simulink model "tous"  (R2025a)
settings: Solver=VariableStepAuto  StartTime=0.0  StopTime=10.0  RelTol=1e-3
undefined symbols (not defined in the file or in its folder): stateSpaceParameters_1
libraries: hdlssclib x12, hdlsllib x10, library_AnalogOut x3, simulink x3
(part 1 of 2)
settings Model: Creator=bensa  LastModifiedBy=bensa

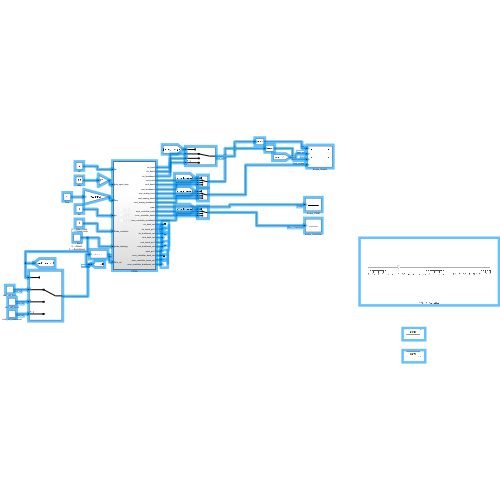
[thumbnail: Simulink's stored preview of the top-level diagram]
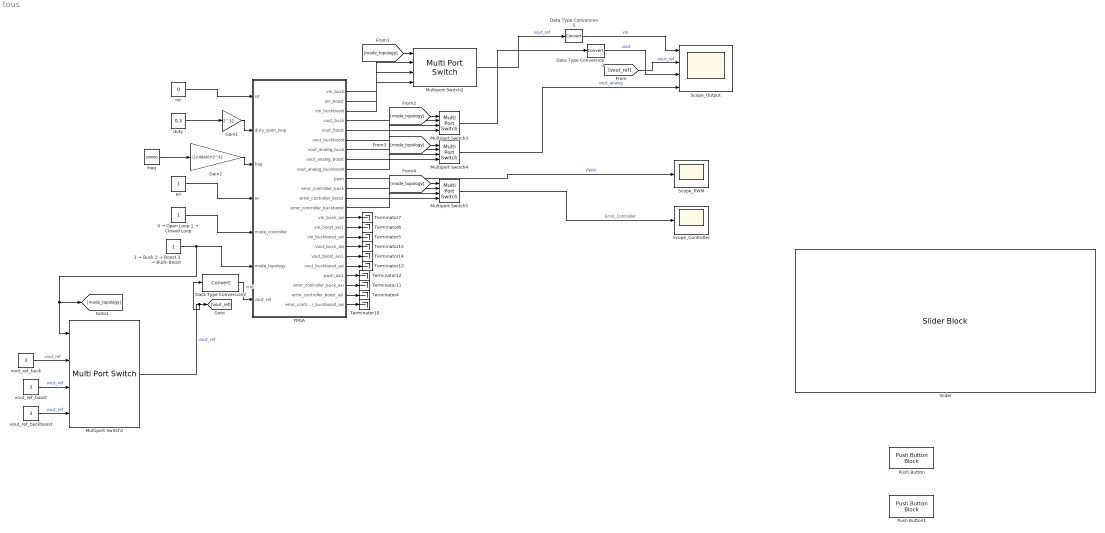
== system tous ==
  0 → Open Loop 1 → Closed Loop : Constant  OutDataTypeStr=uint32  SampleTime=25e-9
  1 → Buck 2 → Boost 3 → Buck-Boost : Constant  OutDataTypeStr=uint32  SampleTime=25e-9
  Data Type Conversion2 : DataTypeConversion  SaturateOnIntegerOverflow=off  RndMeth=Floor
  Data Type Conversion3 : DataTypeConversion  RndMeth=Nearest  SaturateOnIntegerOverflow=off  LockScale=on
  Data Type Conversion5 : DataTypeConversion  RndMeth=Nearest  SaturateOnIntegerOverflow=off  LockScale=on
  FPGA : Subsystem  TreatAsAtomicUnit=on
  Gain1 : Gain  Gain=2^32  OutDataTypeStr=uint32
  Gain2 : Gain  Gain=(1/(40e6))*2^32  OutDataTypeStr=uint32
  Multiport Switch{1..5} (5 alike) : MultiPortSwitch  SaturateOnIntegerOverflow=off  InputSameDT=off
  Push Button : PushButtonBlock  IconOnColor=[0.0, 0.39215686274509803, 0.0]  IconOffColor=[0.0, 1.0, 0.0]
  Push Button1 : PushButtonBlock  IconOnColor=[0.0, 0.39215686274509803, 0.0]  IconOffColor=[0.0, 1.0, 0.0]
  Scope_Controller : Scope
      settings: ActiveDisplayYMinimum=-13.875  ActiveDisplayYMaximum=24.875  DataLoggingVariableName=ScopeData3
  Scope_Output : Scope  NumInputPorts=4
      settings: ActiveDisplayYMinimum=-1.4999999999999996  ActiveDisplayYMaximum=13.5
  Scope_PWM : Scope
      settings: ActiveDisplayYMinimum=-0.62499999999999989  ActiveDisplayYMaximum=5.625
  Slider : SliderBlock  LabelPosition=Bottom  ScaleMax=12
  Terminator{4..7,10..15} (10 alike) : Terminator
  duty : Constant  Value=0.3  OutDataTypeStr=double  SampleTime=25e-9
  en : Constant  OutDataTypeStr=uint32  SampleTime=25e-9
  freq : Constant  Value=100000  SampleTime=25e-9
  rst : Constant  Value=0  OutDataTypeStr=uint32  SampleTime=25e-9
  vout_ref_boost : Constant  Value=3  OutDataTypeStr=double  SampleTime=25e-9
  vout_ref_buck : Constant  Value=3  OutDataTypeStr=double  SampleTime=25e-9
  vout_ref_buckboost : Constant  Value=3  OutDataTypeStr=double  SampleTime=25e-9
  wires:
  duty/1 -> Gain1/1
  [vout_ref] -> Scope_Output/2  "vout_ref"
  FPGA/7(vout_analog_buck) -> Multiport Switch4/2
  FPGA/14(vin_buck_axi) -> Terminator7/1
  FPGA/5(vout_boost) -> Multiport Switch3/3
  FPGA/4(vout_buck) -> Multiport Switch3/2
  0 → Open Loop 1 → Closed Loop/1 -> FPGA/5(mode_controller)
  1 → Buck 2 → Boost 3 → Buck-Boost/1 -> FPGA/6(mode_topology), [mode_topology], Multiport Switch1/1
  FPGA/22(error_controller_boost_axi) -> Terminator4/1
  FPGA/12(error_controller_boost) -> Multiport Switch5/3
  Data Type Conversion3/1 -> Scope_Output/3  "vout"
  FPGA/2(vin_boost) -> Multiport Switch2/3
  FPGA/11(error_controller_buck) -> Multiport Switch5/2
  FPGA/13(error_controller_buckboost) -> Multiport Switch5/4
  vout_ref_buck/1 -> Multiport Switch1/2  "vout_ref"
  FPGA/21(error_controller_buck_axi) -> Terminator11/1
  [mode_topology] -> Multiport Switch2/1
  FPGA/16(vin_buckboost_axi) -> Terminator5/1
  FPGA/10(pwm) -> Scope_PWM/1  "PWM"
  rst/1 -> FPGA/1(rst)
  Multiport Switch4/1 -> Scope_Output/4  "vout_analog"
  FPGA/17(vout_buck_axi) -> Terminator15/1
  FPGA/9(vout_analog_buckboost) -> Multiport Switch4/4
  freq/1 -> Gain2/1
  Multiport Switch5/1 -> Scope_Controller/1  "Error_Controller"
  Multiport Switch2/1 -> Data Type Conversion5/1  "vout_ref"
  FPGA/6(vout_buckboost) -> Multiport Switch3/4
  Gain1/1 -> FPGA/2(duty_open_loop)
  Multiport Switch1/1 -> Data Type Conversion2/1, [vout_ref]  "vout_ref"
  FPGA/23(error_controller_buckboost_axi) -> Terminator10/1
  Data Type Conversion2/1 -> FPGA/7(vout_ref)  "vref"
  [mode_topology] -> Multiport Switch5/1
  vout_ref_buckboost/1 -> Multiport Switch1/4  "vout_ref"
  vout_ref_boost/1 -> Multiport Switch1/3  "vout_ref"
  FPGA/1(vin_buck) -> Multiport Switch2/2
  Data Type Conversion5/1 -> Scope_Output/1  "vin"
  en/1 -> FPGA/4(en)
  FPGA/8(vout_analog_boost) -> Multiport Switch4/3
  [mode_topology] -> Multiport Switch3/1
  FPGA/19(vout_buckboost_axi) -> Terminator13/1
  FPGA/18(vout_boost_axi1) -> Terminator14/1
  Gain2/1 -> FPGA/3(freq)
  Multiport Switch3/1 -> Data Type Conversion3/1
  [mode_topology] -> Multiport Switch4/1
  FPGA/20(pwm_axi1) -> Terminator12/1
  FPGA/3(vin_buckboost) -> Multiport Switch2/4
  FPGA/15(vin_boost_axi1) -> Terminator6/1

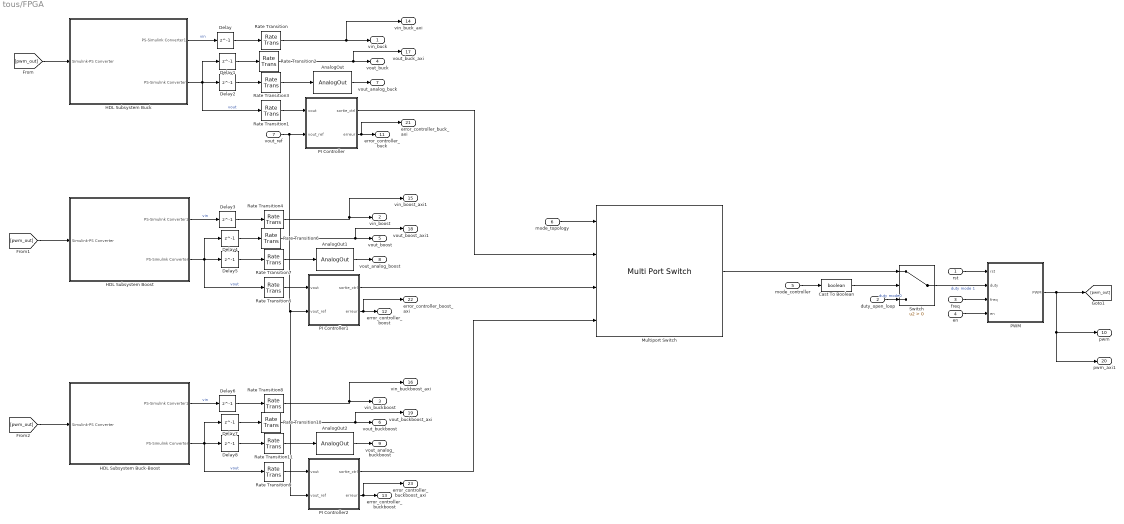
== system tous/FPGA ==
  rst : Inport  OutDataTypeStr=uint32
  duty_open_loop : Inport  Port=2  OutDataTypeStr=uint32
  freq : Inport  Port=3  OutDataTypeStr=uint32
  en : Inport  Port=4  OutDataTypeStr=uint32
  mode_controller : Inport  Port=5  OutDataTypeStr=uint32
  mode_topology : Inport  Port=6
  vout_ref : Inport  Port=7  OutDataTypeStr=uint32
  AnalogOut : library_AnalogOut/AnalogOut  SignalMin=0  SignalMax=12  VoltageMin=0  VoltageMax=4
  AnalogOut1 : library_AnalogOut/AnalogOut  SignalMin=0  SignalMax=12  VoltageMin=0  VoltageMax=4
  AnalogOut2 : library_AnalogOut/AnalogOut  SignalMin=0  SignalMax=12  VoltageMin=0  VoltageMax=4
  Cast To Boolean : DataTypeConversion  OutDataTypeStr=boolean  SaturateOnIntegerOverflow=off  RndMeth=Floor
  Delay{,1..8} (9 alike) : Delay  DelayLength=1
  HDL Subsystem Boost : Subsystem  DataTypeOverride=Off  MinMaxOverflowLogging=MinMaxAndOverflow
  HDL Subsystem Buck : Subsystem  DataTypeOverride=Off  MinMaxOverflowLogging=MinMaxAndOverflow
  HDL Subsystem Buck-Boost : Subsystem  DataTypeOverride=Off  MinMaxOverflowLogging=MinMaxAndOverflow
  Multiport Switch : MultiPortSwitch  SaturateOnIntegerOverflow=off  InputSameDT=off
  PI Controller : Subsystem
  PI Controller1 : Subsystem
  PI Controller2 : Subsystem
  PWM : Subsystem
  Rate Transition{,2..4,6..8,10..11} (9 alike) : RateTransition  OutPortSampleTime=25e-9
  Rate Transition1 : RateTransition
  Rate Transition5 : RateTransition
  Rate Transition9 : RateTransition
  Switch : Switch  Criteria=u2 > Threshold  SaturateOnIntegerOverflow=off  InputSameDT=off
  vin_buck : Outport
  vin_boost : Outport  Port=2
  vin_buckboost : Outport  Port=3
  vout_buck : Outport  Port=4
  vout_boost : Outport  Port=5
  vout_buckboost : Outport  Port=6
  vout_analog_buck : Outport  Port=7
  vout_analog_boost : Outport  Port=8
  vout_analog_buckboost : Outport  Port=9
  pwm : Outport  Port=10
  error_controller_buck : Outport  Port=11
  error_controller_boost : Outport  Port=12
  error_controller_buckboost : Outport  Port=13
  vin_buck_axi : Outport  Port=14
  vin_boost_axi1 : Outport  Port=15
  vin_buckboost_axi : Outport  Port=16
  vout_buck_axi : Outport  Port=17
  vout_boost_axi1 : Outport  Port=18
  vout_buckboost_axi : Outport  Port=19
  pwm_axi1 : Outport  Port=20
  error_controller_buck_axi : Outport  Port=21
  error_controller_boost_axi : Outport  Port=22
  error_controller_buckboost_axi : Outport  Port=23
  wires:
  HDL Subsystem Buck/1(PS-Simulink Converter1) -> Delay/1  "vin"
  HDL Subsystem Buck/2(PS-Simulink Converter) -> Rate Transition1/1, Delay2/1, Delay1/1  "vout"
  Delay1/1 -> Rate Transition2/1
  Delay/1 -> Rate Transition/1
  Rate Transition2/1 -> vout_buck_axi/1, vout_buck/1
  Rate Transition/1 -> vin_buck_axi/1, vin_buck/1
  AnalogOut/1 -> vout_analog_buck/1
  PI Controller/2(erreur) -> error_controller_buck_axi/1, error_controller_buck/1
  Rate Transition1/1 -> PI Controller/1(vout)
  Delay2/1 -> Rate Transition3/1
  Rate Transition3/1 -> AnalogOut/1
  PI Controller/1(sortie_ctrl) -> Multiport Switch/2
  mode_topology/1 -> Multiport Switch/1
  Delay4/1 -> Rate Transition6/1
  Rate Transition7/1 -> AnalogOut1/1
  Delay3/1 -> Rate Transition4/1
  PI Controller1/2(erreur) -> error_controller_boost_axi/1, error_controller_boost/1
  PI Controller1/1(sortie_ctrl) -> Multiport Switch/3
  HDL Subsystem Boost/1(PS-Simulink Converter1) -> Delay3/1  "vin"
  HDL Subsystem Boost/2(PS-Simulink Converter) -> Rate Transition5/1, Delay5/1, Delay4/1  "vout"
  Rate Transition6/1 -> vout_boost_axi1/1, vout_boost/1
  Rate Transition5/1 -> PI Controller1/1(vout)
  Rate Transition4/1 -> vin_boost_axi1/1, vin_boost/1
  Delay5/1 -> Rate Transition7/1
  AnalogOut1/1 -> vout_analog_boost/1
  vout_ref/1 -> PI Controller2/2(vout_ref), PI Controller1/2(vout_ref), PI Controller/2(vout_ref)
  Delay7/1 -> Rate Transition10/1
  Rate Transition11/1 -> AnalogOut2/1
  Delay6/1 -> Rate Transition8/1
  PI Controller2/2(erreur) -> error_controller_buckboost_axi/1, error_controller_buckboost/1
  PI Controller2/1(sortie_ctrl) -> Multiport Switch/4
  HDL Subsystem Buck-Boost/1(PS-Simulink Converter1) -> Delay6/1  "vin"
  HDL Subsystem Buck-Boost/2(PS-Simulink Converter) -> Rate Transition9/1, Delay8/1, Delay7/1  "vout"
  Rate Transition10/1 -> vout_buckboost_axi/1, vout_buckboost/1
  Rate Transition9/1 -> PI Controller2/1(vout)
  Rate Transition8/1 -> vin_buckboost_axi/1, vin_buckboost/1
  Delay8/1 -> Rate Transition11/1
  AnalogOut2/1 -> vout_analog_buckboost/1
  Multiport Switch/1 -> Switch/1
  Switch/1 -> PWM/2(duty)  "duty mode 1"
  duty_open_loop/1 -> Switch/3  "duty mode0"
  freq/1 -> PWM/3(freq)
  rst/1 -> PWM/1(rst)
  en/1 -> PWM/4(en)
  Cast To Boolean/1 -> Switch/2
  mode_controller/1 -> Cast To Boolean/1
  PWM/1(PWM) -> pwm/1, pwm_axi1/1, [pwm_out]
  [pwm_out] -> HDL Subsystem Buck/1(Simulink-PS Converter)
  [pwm_out] -> HDL Subsystem Boost/1(Simulink-PS Converter)
  [pwm_out] -> HDL Subsystem Buck-Boost/1(Simulink-PS Converter)

== system tous/FPGA/HDL Subsystem Boost ==
  Simulink-PS Converter : Inport  OutDataTypeStr=fixdt(0,32,29)
  HDL Algorithm : Subsystem
  Input Concat : Concatenate  NumInputs=1
  Output Demux : Demux  Outputs=2
  Rate Transition2 : RateTransition  Integrity=off  OutPortSampleTimeOpt=Multiple of input port sample time  OutPortSampleTimeMultiple=1/2
  Rate Transition3 : RateTransition  OutPortSampleTimeOpt=Multiple of input port sample time  OutPortSampleTimeMultiple=2
  Rate Transition4 : RateTransition  OutPortSampleTimeOpt=Multiple of input port sample time  OutPortSampleTimeMultiple=2
  Valid Out : Terminator
  PS-Simulink Converter1 : Outport
  PS-Simulink Converter : Outport  Port=2
  wires:
  HDL Algorithm/1(Out1) -> Output Demux/1
  Rate Transition3/1 -> PS-Simulink Converter1/1  "PS-Simulink Converter1"
  HDL Algorithm/2(Valid Out) -> Valid Out/1
  Output Demux/2 -> Rate Transition4/1
  Output Demux/1 -> Rate Transition3/1
  Simulink-PS Converter/1 -> Rate Transition2/1
  Input Concat/1 -> HDL Algorithm/1(In1)
  Rate Transition2/1 -> Input Concat/1
  Rate Transition4/1 -> PS-Simulink Converter/1  "PS-Simulink Converter"

== system tous/FPGA/HDL Subsystem Buck ==
  Simulink-PS Converter : Inport  OutDataTypeStr=fixdt(0,32,29)
  HDL Algorithm : Subsystem
  Input Concat : Concatenate  NumInputs=1
  Output Demux : Demux  Outputs=2
  Rate Transition2 : RateTransition  Integrity=off  OutPortSampleTimeOpt=Multiple of input port sample time  OutPortSampleTimeMultiple=1/2
  Rate Transition3 : RateTransition  OutPortSampleTimeOpt=Multiple of input port sample time  OutPortSampleTimeMultiple=2
  Rate Transition4 : RateTransition  OutPortSampleTimeOpt=Multiple of input port sample time  OutPortSampleTimeMultiple=2
  Valid Out : Terminator
  PS-Simulink Converter1 : Outport
  PS-Simulink Converter : Outport  Port=2
  wires:
  Output Demux/2 -> Rate Transition4/1
  Rate Transition3/1 -> PS-Simulink Converter1/1  "PS-Simulink Converter1"
  HDL Algorithm/2(Valid Out) -> Valid Out/1
  Input Concat/1 -> HDL Algorithm/1(In1)
  Output Demux/1 -> Rate Transition3/1
  Simulink-PS Converter/1 -> Rate Transition2/1
  HDL Algorithm/1(Out1) -> Output Demux/1
  Rate Transition4/1 -> PS-Simulink Converter/1  "PS-Simulink Converter"
  Rate Transition2/1 -> Input Concat/1

== system tous/FPGA/HDL Subsystem Buck-Boost ==
  Simulink-PS Converter : Inport  OutDataTypeStr=fixdt(0,32,29)
  HDL Algorithm : Subsystem
  Input Concat : Concatenate  NumInputs=1
  Output Demux : Demux  Outputs=2
  Rate Transition2 : RateTransition  Integrity=off  OutPortSampleTimeOpt=Multiple of input port sample time  OutPortSampleTimeMultiple=1/2
  Rate Transition3 : RateTransition  OutPortSampleTimeOpt=Multiple of input port sample time  OutPortSampleTimeMultiple=2
  Rate Transition4 : RateTransition  OutPortSampleTimeOpt=Multiple of input port sample time  OutPortSampleTimeMultiple=2
  Valid Out : Terminator
  PS-Simulink Converter1 : Outport
  PS-Simulink Converter : Outport  Port=2
  wires:
  Rate Transition3/1 -> PS-Simulink Converter1/1  "PS-Simulink Converter1"
  Rate Transition2/1 -> Input Concat/1
  Input Concat/1 -> HDL Algorithm/1(In1)
  Simulink-PS Converter/1 -> Rate Transition2/1
  Output Demux/1 -> Rate Transition3/1
  Rate Transition4/1 -> PS-Simulink Converter/1  "PS-Simulink Converter"
  Output Demux/2 -> Rate Transition4/1
  HDL Algorithm/1(Out1) -> Output Demux/1
  HDL Algorithm/2(Valid Out) -> Valid Out/1

== system tous/FPGA/PI Controller ==
  vout : Inport
  vout_ref : Inport  Port=2  OutDataTypeStr=uint32
  Controller : Subsystem
  Data Type Conversion : DataTypeConversion  SaturateOnIntegerOverflow=off  RndMeth=Floor
  Data Type Conversion1 : DataTypeConversion  SaturateOnIntegerOverflow=off  RndMeth=Floor
  Data Type Conversion2 : DataTypeConversion  SaturateOnIntegerOverflow=off  RndMeth=Floor
  Gain3 : Gain  Gain=2^32  OutDataTypeStr=uint32
  ki : Constant  Value=3.07e-80  OutDataTypeStr=double  SampleTime=25e-9
  kp : Constant  Value=3  OutDataTypeStr=double  SampleTime=25e-9
  sortie_ctrl : Outport
  erreur : Outport  Port=2
  wires:
  vout/1 -> Data Type Conversion/1
  Controller/1(sortie_ctrl) -> Gain3/1
  Data Type Conversion1/1 -> Controller/3(kp)
  kp/1 -> Data Type Conversion1/1
  ki/1 -> Data Type Conversion2/1
  vout_ref/1 -> Controller/1(vout_ref)
  Data Type Conversion/1 -> Controller/2(vout)
  Data Type Conversion2/1 -> Controller/4(ki)
  Gain3/1 -> sortie_ctrl/1
  Controller/2(error_ctrl) -> erreur/1

== system tous/FPGA/PI Controller1 ==
  vout : Inport
  vout_ref : Inport  Port=2  OutDataTypeStr=uint32
  Controller : Subsystem
  Data Type Conversion : DataTypeConversion  SaturateOnIntegerOverflow=off  RndMeth=Floor
  Data Type Conversion1 : DataTypeConversion  SaturateOnIntegerOverflow=off  RndMeth=Floor
  Data Type Conversion2 : DataTypeConversion  SaturateOnIntegerOverflow=off  RndMeth=Floor
  Gain3 : Gain  Gain=2^32  OutDataTypeStr=uint32
  ki : Constant  Value=3.07e-80  OutDataTypeStr=double  SampleTime=25e-9
  kp : Constant  Value=3  OutDataTypeStr=double  SampleTime=25e-9
  sortie_ctrl : Outport
  erreur : Outport  Port=2
  wires:
  vout/1 -> Data Type Conversion/1
  Controller/1(sortie_ctrl) -> Gain3/1
  Data Type Conversion1/1 -> Controller/3(kp)
  kp/1 -> Data Type Conversion1/1
  ki/1 -> Data Type Conversion2/1
  vout_ref/1 -> Controller/1(vout_ref)
  Data Type Conversion/1 -> Controller/2(vout)
  Data Type Conversion2/1 -> Controller/4(ki)
  Gain3/1 -> sortie_ctrl/1
  Controller/2(error_ctrl) -> erreur/1

== system tous/FPGA/PI Controller2 ==
  vout : Inport
  vout_ref : Inport  Port=2  OutDataTypeStr=uint32
  Controller : Subsystem
  Data Type Conversion : DataTypeConversion  SaturateOnIntegerOverflow=off  RndMeth=Floor
  Data Type Conversion1 : DataTypeConversion  SaturateOnIntegerOverflow=off  RndMeth=Floor
  Data Type Conversion2 : DataTypeConversion  SaturateOnIntegerOverflow=off  RndMeth=Floor
  Gain3 : Gain  Gain=2^32  OutDataTypeStr=uint32
  ki : Constant  Value=3.07e-80  OutDataTypeStr=double  SampleTime=25e-9
  kp : Constant  Value=3  OutDataTypeStr=double  SampleTime=25e-9
  sortie_ctrl : Outport
  erreur : Outport  Port=2
  wires:
  vout/1 -> Data Type Conversion/1
  Controller/1(sortie_ctrl) -> Gain3/1
  Data Type Conversion1/1 -> Controller/3(kp)
  kp/1 -> Data Type Conversion1/1
  ki/1 -> Data Type Conversion2/1
  vout_ref/1 -> Controller/1(vout_ref)
  Data Type Conversion/1 -> Controller/2(vout)
  Data Type Conversion2/1 -> Controller/4(ki)
  Gain3/1 -> sortie_ctrl/1
  Controller/2(error_ctrl) -> erreur/1

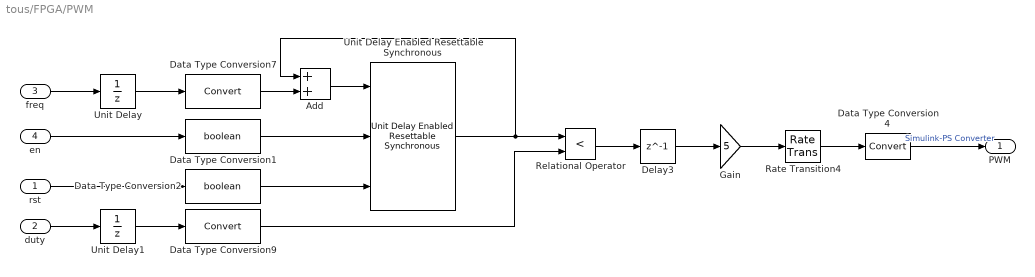
== system tous/FPGA/PWM ==
  rst : Inport  OutDataTypeStr=uint32
  duty : Inport  Port=2  OutDataTypeStr=uint32
  freq : Inport  Port=3  OutDataTypeStr=uint32
  en : Inport  Port=4  OutDataTypeStr=uint32
  Add : Sum  OutDataTypeStr=uint32  AccumDataTypeStr=uint32
  Data Type Conversion1 : DataTypeConversion  OutDataTypeStr=boolean  SaturateOnIntegerOverflow=off  RndMeth=Floor
  Data Type Conversion2 : DataTypeConversion  OutDataTypeStr=boolean  SaturateOnIntegerOverflow=off  RndMeth=Floor
  Data Type Conversion4 : DataTypeConversion  RndMeth=Nearest  SaturateOnIntegerOverflow=off
  Data Type Conversion7 : DataTypeConversion  SaturateOnIntegerOverflow=off  RndMeth=Floor
  Data Type Conversion9 : DataTypeConversion  SaturateOnIntegerOverflow=off  RndMeth=Floor
  Delay3 : Delay  DelayLength=1
  Gain : Gain  Gain=5
  Rate Transition4 : RateTransition  OutPortSampleTime=5e-08
  Relational Operator : RelationalOperator  Operator=<  OutDataTypeStr=boolean  RndMeth=Simplest  InputSameDT=off
  Unit Delay : UnitDelay  SampleTime=-1  HasFrameUpgradeWarning=on
  Unit Delay Enabled Resettable Synchronous : hdlsllib/Discrete/Unit Delay Enabled Resettable Synchronous  InitialCondition=0.0  SampleTime=-1
  Unit Delay1 : UnitDelay  SampleTime=-1  HasFrameUpgradeWarning=on
  PWM : Outport
  wires:
  Rate Transition4/1 -> Data Type Conversion4/1
  en/1 -> Data Type Conversion1/1
  Data Type Conversion1/1 -> Unit Delay Enabled Resettable Synchronous/2
  Unit Delay/1 -> Data Type Conversion7/1
  Data Type Conversion7/1 -> Add/2
  Gain/1 -> Rate Transition4/1
  Delay3/1 -> Gain/1
  Data Type Conversion2/1 -> Unit Delay Enabled Resettable Synchronous/3
  Add/1 -> Unit Delay Enabled Resettable Synchronous/1
  freq/1 -> Unit Delay/1
  Unit Delay Enabled Resettable Synchronous/1 -> Add/1, Relational Operator/1
  Unit Delay1/1 -> Data Type Conversion9/1
  rst/1 -> Data Type Conversion2/1
  Data Type Conversion9/1 -> Relational Operator/2
  Relational Operator/1 -> Delay3/1
  duty/1 -> Unit Delay1/1
  Data Type Conversion4/1 -> PWM/1  "Simulink-PS Converter"

== system tous/FPGA/HDL Subsystem Boost/HDL Algorithm ==
  In1 : Inport  OutDataTypeStr=fixdt(0,32,29)
  Delay : Delay  DelayLength=1
  Delay1 : Delay
  Mode Iteration Manager : Subsystem
  Mode Selection : Subsystem
  Output : Subsystem
  State Delay : Delay  DelayLength=1  InitialCondition=single(stateSpaceParameters_1.X0)
  State Update : Subsystem
  Out1 : Outport  VectorParamsAs1DForOutWhenUnconnected=off
  Valid Out : Outport  Port=2  VectorParamsAs1DForOutWhenUnconnected=off
  wires:
  In1/1 -> Mode Selection/1(In1), Delay1/1, State Update/1(In1)
  Delay1/1 -> Output/1(In1)
  State Update/1(State Out) -> State Delay/1
  Mode Selection/1(Out1) -> Mode Iteration Manager/2(In2)
  State Delay/1 -> Mode Iteration Manager/1(In1), Mode Selection/2(In2)
  Delay/1 -> Output/3(Sel)
  Mode Iteration Manager/1(Out1) -> State Update/2(State), Output/2(State)
  Mode Selection/2(Out2) -> Delay/1
  Mode Iteration Manager/2(Out2) -> State Update/3(Sel)
  Mode Iteration Manager/3(Valid Out) -> Valid Out/1
  Output/1(Out1) -> Out1/1

== system tous/FPGA/HDL Subsystem Buck/HDL Algorithm ==
  In1 : Inport  OutDataTypeStr=fixdt(0,32,29)
  Delay : Delay  DelayLength=1
  Delay1 : Delay
  Mode Iteration Manager : Subsystem
  Mode Selection : Subsystem
  Output : Subsystem
  State Delay : Delay  DelayLength=1  InitialCondition=single(stateSpaceParameters_1.X0)
  State Update : Subsystem
  Out1 : Outport  VectorParamsAs1DForOutWhenUnconnected=off
  Valid Out : Outport  Port=2  VectorParamsAs1DForOutWhenUnconnected=off
  wires:
  In1/1 -> Mode Selection/1(In1), Delay1/1, State Update/1(In1)
  State Update/1(State Out) -> State Delay/1
  Delay1/1 -> Output/1(In1)
  Mode Selection/2(Out2) -> Delay/1
  State Delay/1 -> Mode Iteration Manager/1(In1), Mode Selection/2(In2)
  Mode Selection/1(Out1) -> Mode Iteration Manager/2(In2)
  Delay/1 -> Output/3(Sel)
  Mode Iteration Manager/1(Out1) -> State Update/2(State), Output/2(State)
  Mode Iteration Manager/2(Out2) -> State Update/3(Sel)
  Mode Iteration Manager/3(Valid Out) -> Valid Out/1
  Output/1(Out1) -> Out1/1

== system tous/FPGA/HDL Subsystem Buck-Boost/HDL Algorithm ==
  In1 : Inport  OutDataTypeStr=fixdt(0,32,29)
  Delay : Delay  DelayLength=1
  Delay1 : Delay
  Mode Iteration Manager : Subsystem
  Mode Selection : Subsystem
  Output : Subsystem
  State Delay : Delay  DelayLength=1  InitialCondition=single(stateSpaceParameters_1.X0)
  State Update : Subsystem
  Out1 : Outport  VectorParamsAs1DForOutWhenUnconnected=off
  Valid Out : Outport  Port=2  VectorParamsAs1DForOutWhenUnconnected=off
  wires:
  In1/1 -> Mode Selection/1(In1), Delay1/1, State Update/1(In1)
  Delay/1 -> Output/3(Sel)
  Mode Selection/1(Out1) -> Mode Iteration Manager/2(In2)
  State Update/1(State Out) -> State Delay/1
  Delay1/1 -> Output/1(In1)
  Mode Selection/2(Out2) -> Delay/1
  Mode Iteration Manager/1(Out1) -> State Update/2(State), Output/2(State)
  State Delay/1 -> Mode Iteration Manager/1(In1), Mode Selection/2(In2)
  Mode Iteration Manager/2(Out2) -> State Update/3(Sel)
  Mode Iteration Manager/3(Valid Out) -> Valid Out/1
  Output/1(Out1) -> Out1/1

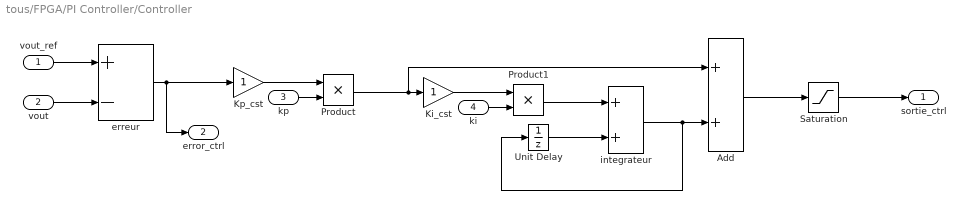
== system tous/FPGA/PI Controller/Controller ==
  vout_ref : Inport
  vout : Inport  Port=2
  kp : Inport  Port=3
  ki : Inport  Port=4
  Add : Sum  OutDataTypeStr=fixdt(1,32,25)  AccumDataTypeStr=fixdt(1,32,25)
  Ki_cst : Gain  OutDataTypeStr=fixdt(1,32,25)
  Kp_cst : Gain  OutDataTypeStr=fixdt(1,32,25)
  Product : Product
  Product1 : Product
  Saturation : Saturate  UpperLimit=0.95  LowerLimit=0.05  LinearizeAsGain=off
  Unit Delay : UnitDelay  SampleTime=-1  HasFrameUpgradeWarning=on
  erreur : Sum  Inputs=+-  OutDataTypeStr=fixdt(1,32,25)  AccumDataTypeStr=fixdt(1,32,25)
  integrateur : Sum  OutDataTypeStr=fixdt(1,32,25)  AccumDataTypeStr=fixdt(1,32,25)
  sortie_ctrl : Outport
  error_ctrl : Outport  Port=2
  wires:
  vout/1 -> erreur/2
  vout_ref/1 -> erreur/1
  integrateur/1 -> Unit Delay/1, Add/2
  erreur/1 -> error_ctrl/1, Kp_cst/1
  ki/1 -> Product1/2
  Ki_cst/1 -> Product1/1
  Kp_cst/1 -> Product/1
  Product/1 -> Add/1, Ki_cst/1
  kp/1 -> Product/2
  Product1/1 -> integrateur/1
  Add/1 -> Saturation/1
  Saturation/1 -> sortie_ctrl/1
  Unit Delay/1 -> integrateur/2

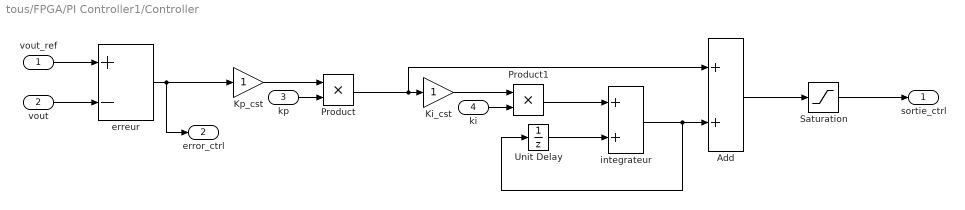
== system tous/FPGA/PI Controller1/Controller ==
  vout_ref : Inport
  vout : Inport  Port=2
  kp : Inport  Port=3
  ki : Inport  Port=4
  Add : Sum  OutDataTypeStr=fixdt(1,32,25)  AccumDataTypeStr=fixdt(1,32,25)
  Ki_cst : Gain  OutDataTypeStr=fixdt(1,32,25)
  Kp_cst : Gain  OutDataTypeStr=fixdt(1,32,25)
  Product : Product
  Product1 : Product
  Saturation : Saturate  UpperLimit=0.95  LowerLimit=0.05  LinearizeAsGain=off
  Unit Delay : UnitDelay  SampleTime=-1  HasFrameUpgradeWarning=on
  erreur : Sum  Inputs=+-  OutDataTypeStr=fixdt(1,32,25)  AccumDataTypeStr=fixdt(1,32,25)
  integrateur : Sum  OutDataTypeStr=fixdt(1,32,25)  AccumDataTypeStr=fixdt(1,32,25)
  sortie_ctrl : Outport
  error_ctrl : Outport  Port=2
  wires:
  vout/1 -> erreur/2
  vout_ref/1 -> erreur/1
  integrateur/1 -> Unit Delay/1, Add/2
  erreur/1 -> error_ctrl/1, Kp_cst/1
  ki/1 -> Product1/2
  Ki_cst/1 -> Product1/1
  Kp_cst/1 -> Product/1
  Product/1 -> Add/1, Ki_cst/1
  kp/1 -> Product/2
  Product1/1 -> integrateur/1
  Add/1 -> Saturation/1
  Saturation/1 -> sortie_ctrl/1
  Unit Delay/1 -> integrateur/2

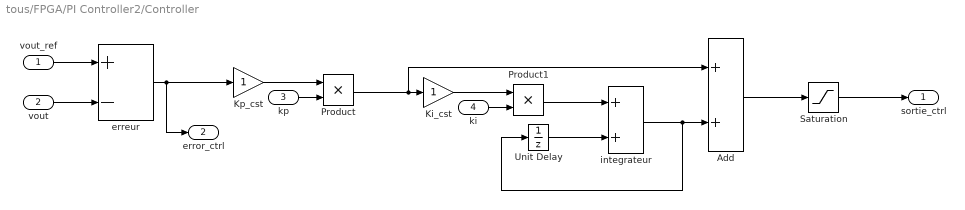
== system tous/FPGA/PI Controller2/Controller ==
  vout_ref : Inport
  vout : Inport  Port=2
  kp : Inport  Port=3
  ki : Inport  Port=4
  Add : Sum  OutDataTypeStr=fixdt(1,32,25)  AccumDataTypeStr=fixdt(1,32,25)
  Ki_cst : Gain  OutDataTypeStr=fixdt(1,32,25)
  Kp_cst : Gain  OutDataTypeStr=fixdt(1,32,25)
  Product : Product
  Product1 : Product
  Saturation : Saturate  UpperLimit=0.95  LowerLimit=0.05  LinearizeAsGain=off
  Unit Delay : UnitDelay  SampleTime=-1  HasFrameUpgradeWarning=on
  erreur : Sum  Inputs=+-  OutDataTypeStr=fixdt(1,32,25)  AccumDataTypeStr=fixdt(1,32,25)
  integrateur : Sum  OutDataTypeStr=fixdt(1,32,25)  AccumDataTypeStr=fixdt(1,32,25)
  sortie_ctrl : Outport
  error_ctrl : Outport  Port=2
  wires:
  vout/1 -> erreur/2
  vout_ref/1 -> erreur/1
  integrateur/1 -> Unit Delay/1, Add/2
  erreur/1 -> error_ctrl/1, Kp_cst/1
  ki/1 -> Product1/2
  Ki_cst/1 -> Product1/1
  Kp_cst/1 -> Product/1
  Product/1 -> Add/1, Ki_cst/1
  kp/1 -> Product/2
  Product1/1 -> integrateur/1
  Add/1 -> Saturation/1
  Saturation/1 -> sortie_ctrl/1
  Unit Delay/1 -> integrateur/2

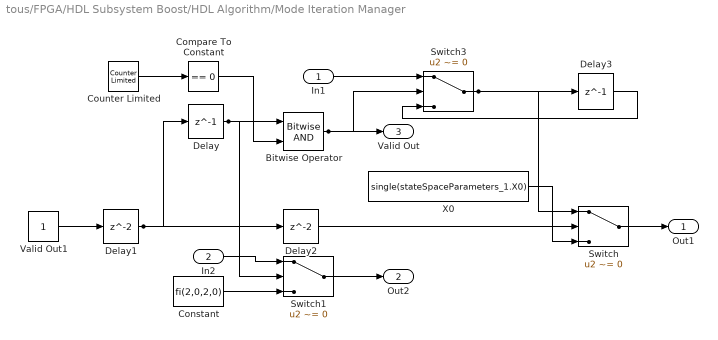
== system tous/FPGA/HDL Subsystem Boost/HDL Algorithm/Mode Iteration Manager ==
  In1 : Inport  LockScale=on
  In2 : Inport  Port=2  OutDataTypeStr=fixdt(0,2,0)  LockScale=on
  Bitwise Operator : simulink/Logic and Bit Operations/Bitwise Operator  logicop=AND  UseBitMask=off  NumInputPorts=2  BitMask=bin2dec('11011001')  BitMaskRealWorld=Stored Integer
      settings: LibrarySourceBlock=|
      | hdlsllib/Logic and Bit
      | Operations/Bitwise
      | Operator
  Compare To Constant : hdlsllib/Logic and Bit Operations/Compare To Constant  relop===  const=0  OutDataTypeStr=boolean
  Constant : Constant  Value=fi(2,0,2,0)  SampleTime=2.5e-08  LockScale=on
  Counter Limited : hdlsllib/Sources/Counter Limited  uplimit=1  tsamp=-1
  Delay : Delay  DelayLength=1
  Delay1 : Delay
  Delay2 : Delay
  Delay3 : Delay  DelayLength=1
  Switch : Switch  Criteria=u2 ~= 0  OutDataTypeStr=fixdt(1,32,27)  SaturateOnIntegerOverflow=off  InputSameDT=off
  Switch1 : Switch  Criteria=u2 ~= 0  SaturateOnIntegerOverflow=off  InputSameDT=off  OutDataTypeStr=Inherit: Same as first input
      settings: LockScale=on
  Switch3 : Switch  Criteria=u2 ~= 0  OutDataTypeStr=fixdt(1,32,27)  SaturateOnIntegerOverflow=off  InputSameDT=off
  Valid Out1 : Constant  OutDataTypeStr=boolean  SampleTime=2.5e-08
  X0 : Constant  Value=single(stateSpaceParameters_1.X0)  OutDataTypeStr=fixdt(0,32,29)  SampleTime=2.5e-08
  Out1 : Outport  OutDataTypeStr=fixdt(1,32,27)  VectorParamsAs1DForOutWhenUnconnected=off
  Out2 : Outport  Port=2  VectorParamsAs1DForOutWhenUnconnected=off
  Valid Out : Outport  Port=3  VectorParamsAs1DForOutWhenUnconnected=off
  wires:
  Constant/1 -> Switch1/3
  Valid Out1/1 -> Delay1/1
  Counter Limited/1 -> Compare To Constant/1
  Delay/1 -> Bitwise Operator/1, Switch1/2
  Delay1/1 -> Delay2/1, Delay/1
  Compare To Constant/1 -> Bitwise Operator/2
  In2/1 -> Switch1/1
  Delay3/1 -> Switch3/3
  In1/1 -> Switch3/1
  Bitwise Operator/1 -> Valid Out/1, Switch3/2
  Delay2/1 -> Switch/2
  Switch/1 -> Out1/1
  Switch1/1 -> Out2/1
  Switch3/1 -> Delay3/1, Switch/1
  X0/1 -> Switch/3

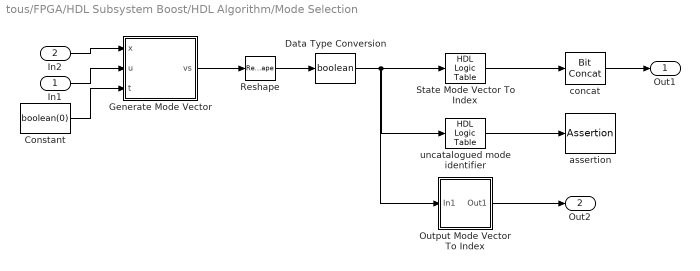
== system tous/FPGA/HDL Subsystem Boost/HDL Algorithm/Mode Selection ==
  In1 : Inport  OutDataTypeStr=fixdt(0,32,29)
  In2 : Inport  Port=2  LockScale=on
  Constant : Constant  Value=boolean(0)  SampleTime=2.5e-08
  Data Type Conversion : DataTypeConversion  OutDataTypeStr=boolean  RndMeth=Nearest  SaturateOnIntegerOverflow=off
  Generate Mode Vector : Subsystem  TreatAsAtomicUnit=on  Variant=on
  Output Mode Vector To Index : Subsystem
  Reshape : Reshape
  State Mode Vector To Index : hdlssclib/HDL Logic Table  InputTable=stateSpaceParameters_1.logicTableInput  OutputTable=stateSpaceParameters_1.logicTableOutput
  assertion : Assertion  StopWhenAssertionFail=off
  concat : hdlsllib/Logic and Bit Operations/Bit Concat  numInputs=1
  uncatalogued mode identifier : hdlssclib/HDL Logic Table  InputTable=stateSpaceParameters_1.logicTableInput  OutputTable=ones(size(stateSpaceParameters_1.logicTableOutput,1),1)
  Out1 : Outport  VectorParamsAs1DForOutWhenUnconnected=off  LockScale=on
  Out2 : Outport  Port=2  VectorParamsAs1DForOutWhenUnconnected=off
  wires:
  Output Mode Vector To Index/1(Out1) -> Out2/1
  State Mode Vector To Index/1 -> concat/1
  Reshape/1 -> Data Type Conversion/1
  Data Type Conversion/1 -> uncatalogued mode identifier/1, State Mode Vector To Index/1, Output Mode Vector To Index/1(In1)
  uncatalogued mode identifier/1 -> assertion/1
  concat/1 -> Out1/1
  In2/1 -> Generate Mode Vector/1(x)
  In1/1 -> Generate Mode Vector/2(u)
  Constant/1 -> Generate Mode Vector/3(t)
  Generate Mode Vector/1(vs) -> Reshape/1

== system tous/FPGA/HDL Subsystem Boost/HDL Algorithm/Output ==
  In1 : Inport  OutDataTypeStr=fixdt(0,32,29)
  State : Inport  Port=2  OutDataTypeStr=fixdt(1,32,27)
  Sel : Inport  Port=3  LockScale=on
  Bias : Subsystem
  Multiply Input : Terminator
  Mux : Mux  Inputs=2
  Output Update : hdlssclib/NFPSparseConstMultiply  MatrixSource=Dialog  constMatrix=fi((([stateSpaceParameters_1.Cd repmat(eye(2),[1,1,1])])),0,32,31)  MatrixType=fixdt(0,32,31)  MatrixSize=[1 1]  ColumnIndices=[1]  RowIndices=[1]  PropDataType=fixdt(1,32,27)  defWL=32
  Out1 : Outport  VectorParamsAs1DForOutWhenUnconnected=off
  wires:
  Sel/1 -> Output Update/2, Bias/1(Sel)
  Mux/1 -> Output Update/1
  In1/1 -> Multiply Input/1
  Bias/1(Out1) -> Mux/2
  State/1 -> Mux/1
  Output Update/1 -> Out1/1

== system tous/FPGA/HDL Subsystem Boost/HDL Algorithm/State Update ==
  In1 : Inport  OutDataTypeStr=fixdt(0,32,29)
  State : Inport  Port=2  OutDataTypeStr=fixdt(1,32,27)
  Sel : Inport  Port=3  LockScale=on
  Bias : Subsystem
  Multiply Input : Terminator
  Mux : Mux  Inputs=2
  State Update : hdlssclib/NFPSparseConstMultiply  MatrixSource=Dialog  constMatrix=fi((([stateSpaceParameters_1.Ad repmat(eye(4),[1,1,4])])),1,32,20)  MatrixType=fixdt(1,32,20)  MatrixSize=[1 1]  ColumnIndices=[1]  RowIndices=[1]  PropDataType=fixdt(1,32,17)  defWL=32
  State Out : Outport  VectorParamsAs1DForOutWhenUnconnected=off
  wires:
  Bias/1(Out1) -> Mux/2
  Sel/1 -> State Update/2, Bias/1(Sel)
  State Update/1 -> State Out/1
  In1/1 -> Multiply Input/1
  Mux/1 -> State Update/1
  State/1 -> Mux/1

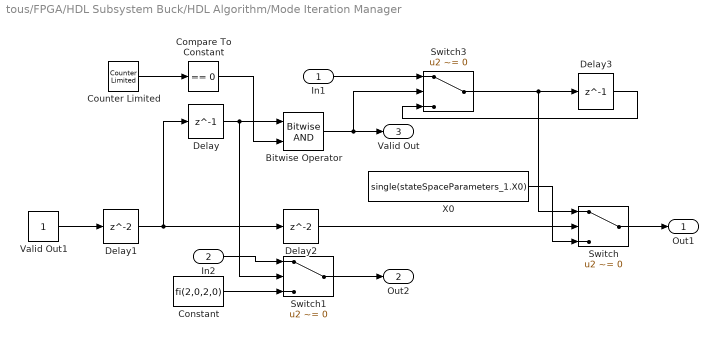
== system tous/FPGA/HDL Subsystem Buck/HDL Algorithm/Mode Iteration Manager ==
  In1 : Inport  LockScale=on
  In2 : Inport  Port=2  OutDataTypeStr=fixdt(0,2,0)  LockScale=on
  Bitwise Operator : simulink/Logic and Bit Operations/Bitwise Operator  logicop=AND  UseBitMask=off  NumInputPorts=2  BitMask=bin2dec('11011001')  BitMaskRealWorld=Stored Integer
      settings: LibrarySourceBlock=|
      | hdlsllib/Logic and Bit
      | Operations/Bitwise
      | Operator
  Compare To Constant : hdlsllib/Logic and Bit Operations/Compare To Constant  relop===  const=0  OutDataTypeStr=boolean
  Constant : Constant  Value=fi(2,0,2,0)  SampleTime=2.5e-08  LockScale=on
  Counter Limited : hdlsllib/Sources/Counter Limited  uplimit=1  tsamp=-1
  Delay : Delay  DelayLength=1
  Delay1 : Delay
  Delay2 : Delay
  Delay3 : Delay  DelayLength=1
  Switch : Switch  Criteria=u2 ~= 0  OutDataTypeStr=fixdt(1,32,24)  SaturateOnIntegerOverflow=off  InputSameDT=off
  Switch1 : Switch  Criteria=u2 ~= 0  SaturateOnIntegerOverflow=off  InputSameDT=off  OutDataTypeStr=Inherit: Same as first input
      settings: LockScale=on
  Switch3 : Switch  Criteria=u2 ~= 0  OutDataTypeStr=fixdt(1,32,27)  SaturateOnIntegerOverflow=off  InputSameDT=off
  Valid Out1 : Constant  OutDataTypeStr=boolean  SampleTime=2.5e-08
  X0 : Constant  Value=single(stateSpaceParameters_1.X0)  OutDataTypeStr=fixdt(1,32,27)  SampleTime=2.5e-08
  Out1 : Outport  OutDataTypeStr=fixdt(1,32,24)  VectorParamsAs1DForOutWhenUnconnected=off
  Out2 : Outport  Port=2  VectorParamsAs1DForOutWhenUnconnected=off
  Valid Out : Outport  Port=3  VectorParamsAs1DForOutWhenUnconnected=off
  wires:
  In2/1 -> Switch1/1
  Valid Out1/1 -> Delay1/1
  In1/1 -> Switch3/1
  Counter Limited/1 -> Compare To Constant/1
  Delay/1 -> Switch1/2, Bitwise Operator/1
  Switch3/1 -> Delay3/1, Switch/1
  Delay1/1 -> Delay2/1, Delay/1
  Compare To Constant/1 -> Bitwise Operator/2
  Constant/1 -> Switch1/3
  Bitwise Operator/1 -> Valid Out/1, Switch3/2
  Delay2/1 -> Switch/2
  Switch1/1 -> Out2/1
  X0/1 -> Switch/3
  Delay3/1 -> Switch3/3
  Switch/1 -> Out1/1

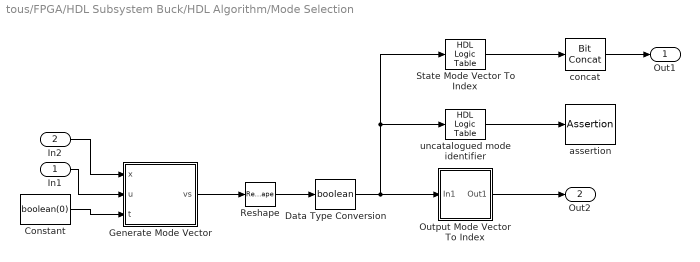
== system tous/FPGA/HDL Subsystem Buck/HDL Algorithm/Mode Selection ==
  In1 : Inport  OutDataTypeStr=fixdt(0,32,29)
  In2 : Inport  Port=2  LockScale=on
  Constant : Constant  Value=boolean(0)  SampleTime=2.5e-08
  Data Type Conversion : DataTypeConversion  OutDataTypeStr=boolean  RndMeth=Nearest  SaturateOnIntegerOverflow=off
  Generate Mode Vector : Subsystem  TreatAsAtomicUnit=on  Variant=on
  Output Mode Vector To Index : Subsystem
  Reshape : Reshape
  State Mode Vector To Index : hdlssclib/HDL Logic Table  InputTable=stateSpaceParameters_1.logicTableInput  OutputTable=stateSpaceParameters_1.logicTableOutput
  assertion : Assertion  StopWhenAssertionFail=off
  concat : hdlsllib/Logic and Bit Operations/Bit Concat  numInputs=1
  uncatalogued mode identifier : hdlssclib/HDL Logic Table  InputTable=stateSpaceParameters_1.logicTableInput  OutputTable=ones(size(stateSpaceParameters_1.logicTableOutput,1),1)
  Out1 : Outport  VectorParamsAs1DForOutWhenUnconnected=off  LockScale=on
  Out2 : Outport  Port=2  VectorParamsAs1DForOutWhenUnconnected=off
  wires:
  uncatalogued mode identifier/1 -> assertion/1
  Reshape/1 -> Data Type Conversion/1
  State Mode Vector To Index/1 -> concat/1
  Data Type Conversion/1 -> uncatalogued mode identifier/1, State Mode Vector To Index/1, Output Mode Vector To Index/1(In1)
  Output Mode Vector To Index/1(Out1) -> Out2/1
  concat/1 -> Out1/1
  In2/1 -> Generate Mode Vector/1(x)
  In1/1 -> Generate Mode Vector/2(u)
  Constant/1 -> Generate Mode Vector/3(t)
  Generate Mode Vector/1(vs) -> Reshape/1

== system tous/FPGA/HDL Subsystem Buck/HDL Algorithm/Output ==
  In1 : Inport  OutDataTypeStr=fixdt(0,32,29)
  State : Inport  Port=2  OutDataTypeStr=fixdt(1,32,24)
  Sel : Inport  Port=3  LockScale=on
  Bias : Subsystem
  Multiply Input : Terminator
  Mux : Mux  Inputs=2
  Output Update : hdlssclib/NFPSparseConstMultiply  MatrixSource=Dialog  constMatrix=fi((([stateSpaceParameters_1.Cd repmat(eye(2),[1,1,1])])),1,32,30)  MatrixType=fixdt(1,32,30)  MatrixSize=[1 1]  ColumnIndices=[1]  RowIndices=[1]  PropDataType=fixdt(1,32,27)  defWL=32
  Out1 : Outport  VectorParamsAs1DForOutWhenUnconnected=off
  wires:
  Sel/1 -> Output Update/2, Bias/1(Sel)
  In1/1 -> Multiply Input/1
  State/1 -> Mux/1
  Bias/1(Out1) -> Mux/2
  Mux/1 -> Output Update/1
  Output Update/1 -> Out1/1

== system tous/FPGA/HDL Subsystem Buck/HDL Algorithm/State Update ==
  In1 : Inport  OutDataTypeStr=fixdt(0,32,29)
  State : Inport  Port=2  OutDataTypeStr=fixdt(1,32,24)
  Sel : Inport  Port=3  LockScale=on
  Bias : Subsystem
  Multiply Input : Terminator
  Mux : Mux  Inputs=2
  State Update : hdlssclib/NFPSparseConstMultiply  MatrixSource=Dialog  constMatrix=fi((([stateSpaceParameters_1.Ad repmat(eye(5),[1,1,4])])),1,32,20)  MatrixType=fixdt(1,32,20)  MatrixSize=[1 1]  ColumnIndices=[1]  RowIndices=[1]  PropDataType=fixdt(1,32,18)  defWL=32
  State Out : Outport  VectorParamsAs1DForOutWhenUnconnected=off
  wires:
  Sel/1 -> State Update/2, Bias/1(Sel)
  In1/1 -> Multiply Input/1
  State/1 -> Mux/1
  Mux/1 -> State Update/1
  Bias/1(Out1) -> Mux/2
  State Update/1 -> State Out/1

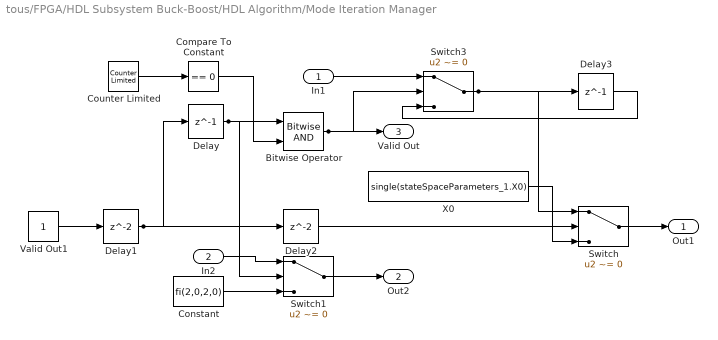
== system tous/FPGA/HDL Subsystem Buck-Boost/HDL Algorithm/Mode Iteration Manager ==
  In1 : Inport  LockScale=on
  In2 : Inport  Port=2  OutDataTypeStr=fixdt(0,2,0)  LockScale=on
  Bitwise Operator : simulink/Logic and Bit Operations/Bitwise Operator  logicop=AND  UseBitMask=off  NumInputPorts=2  BitMask=bin2dec('11011001')  BitMaskRealWorld=Stored Integer
      settings: LibrarySourceBlock=|
      | hdlsllib/Logic and Bit
      | Operations/Bitwise
      | Operator
  Compare To Constant : hdlsllib/Logic and Bit Operations/Compare To Constant  relop===  const=0  OutDataTypeStr=boolean
  Constant : Constant  Value=fi(2,0,2,0)  SampleTime=2.5e-08  LockScale=on
  Counter Limited : hdlsllib/Sources/Counter Limited  uplimit=1  tsamp=-1
  Delay : Delay  DelayLength=1
  Delay1 : Delay
  Delay2 : Delay
  Delay3 : Delay  DelayLength=1
  Switch : Switch  Criteria=u2 ~= 0  OutDataTypeStr=fixdt(1,32,25)  SaturateOnIntegerOverflow=off  InputSameDT=off
  Switch1 : Switch  Criteria=u2 ~= 0  SaturateOnIntegerOverflow=off  InputSameDT=off  OutDataTypeStr=Inherit: Same as first input
      settings: LockScale=on
  Switch3 : Switch  Criteria=u2 ~= 0  OutDataTypeStr=fixdt(1,32,28)  SaturateOnIntegerOverflow=off  InputSameDT=off
  Valid Out1 : Constant  OutDataTypeStr=boolean  SampleTime=2.5e-08
  X0 : Constant  Value=single(stateSpaceParameters_1.X0)  OutDataTypeStr=fixdt(0,32,29)  SampleTime=2.5e-08
  Out1 : Outport  OutDataTypeStr=fixdt(1,32,25)  VectorParamsAs1DForOutWhenUnconnected=off
  Out2 : Outport  Port=2  VectorParamsAs1DForOutWhenUnconnected=off
  Valid Out : Outport  Port=3  VectorParamsAs1DForOutWhenUnconnected=off
  wires:
  Counter Limited/1 -> Compare To Constant/1
  Valid Out1/1 -> Delay1/1
  Delay1/1 -> Delay2/1, Delay/1
  Compare To Constant/1 -> Bitwise Operator/2
  Delay/1 -> Switch1/2, Bitwise Operator/1
  Bitwise Operator/1 -> Valid Out/1, Switch3/2
  In2/1 -> Switch1/1
  In1/1 -> Switch3/1
  Constant/1 -> Switch1/3
  Delay2/1 -> Switch/2
  Switch1/1 -> Out2/1
  Switch3/1 -> Delay3/1, Switch/1
  X0/1 -> Switch/3
  Delay3/1 -> Switch3/3
  Switch/1 -> Out1/1

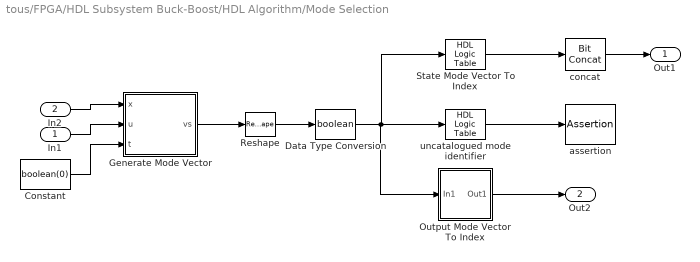
== system tous/FPGA/HDL Subsystem Buck-Boost/HDL Algorithm/Mode Selection ==
  In1 : Inport  OutDataTypeStr=fixdt(0,32,29)
  In2 : Inport  Port=2  LockScale=on
  Constant : Constant  Value=boolean(0)  SampleTime=2.5e-08
  Data Type Conversion : DataTypeConversion  OutDataTypeStr=boolean  RndMeth=Nearest  SaturateOnIntegerOverflow=off
  Generate Mode Vector : Subsystem  TreatAsAtomicUnit=on  Variant=on
  Output Mode Vector To Index : Subsystem
  Reshape : Reshape
  State Mode Vector To Index : hdlssclib/HDL Logic Table  InputTable=stateSpaceParameters_1.logicTableInput  OutputTable=stateSpaceParameters_1.logicTableOutput
  assertion : Assertion  StopWhenAssertionFail=off
  concat : hdlsllib/Logic and Bit Operations/Bit Concat  numInputs=1
  uncatalogued mode identifier : hdlssclib/HDL Logic Table  InputTable=stateSpaceParameters_1.logicTableInput  OutputTable=ones(size(stateSpaceParameters_1.logicTableOutput,1),1)
  Out1 : Outport  VectorParamsAs1DForOutWhenUnconnected=off  LockScale=on
  Out2 : Outport  Port=2  VectorParamsAs1DForOutWhenUnconnected=off
  wires:
  Data Type Conversion/1 -> State Mode Vector To Index/1, uncatalogued mode identifier/1, Output Mode Vector To Index/1(In1)
  State Mode Vector To Index/1 -> concat/1
  Reshape/1 -> Data Type Conversion/1
  uncatalogued mode identifier/1 -> assertion/1
  Output Mode Vector To Index/1(Out1) -> Out2/1
  concat/1 -> Out1/1
  In2/1 -> Generate Mode Vector/1(x)
  In1/1 -> Generate Mode Vector/2(u)
  Constant/1 -> Generate Mode Vector/3(t)
  Generate Mode Vector/1(vs) -> Reshape/1

== system tous/FPGA/HDL Subsystem Buck-Boost/HDL Algorithm/Output ==
  In1 : Inport  OutDataTypeStr=fixdt(0,32,29)
  State : Inport  Port=2  OutDataTypeStr=fixdt(1,32,25)
  Sel : Inport  Port=3  LockScale=on
  Bias : Subsystem
  Multiply Input : Terminator
  Mux : Mux  Inputs=2
  Output Update : hdlssclib/NFPSparseConstMultiply  MatrixSource=Dialog  constMatrix=fi((([stateSpaceParameters_1.Cd repmat(eye(2),[1,1,1])])),0,32,31)  MatrixType=fixdt(0,32,31)  MatrixSize=[1 1]  ColumnIndices=[1]  RowIndices=[1]  PropDataType=fixdt(1,32,28)  defWL=32
  Out1 : Outport  VectorParamsAs1DForOutWhenUnconnected=off
  wires:
  Sel/1 -> Output Update/2, Bias/1(Sel)
  In1/1 -> Multiply Input/1
  State/1 -> Mux/1
  Bias/1(Out1) -> Mux/2
  Mux/1 -> Output Update/1
  Output Update/1 -> Out1/1

== system tous/FPGA/HDL Subsystem Buck-Boost/HDL Algorithm/State Update ==
  In1 : Inport  OutDataTypeStr=fixdt(0,32,29)
  State : Inport  Port=2  OutDataTypeStr=fixdt(1,32,25)
  Sel : Inport  Port=3  LockScale=on
  Bias : Subsystem
  Multiply Input : Terminator
  Mux : Mux  Inputs=2
  State Update : hdlssclib/NFPSparseConstMultiply  MatrixSource=Dialog  constMatrix=fi((([stateSpaceParameters_1.Ad repmat(eye(4),[1,1,4])])),1,32,20)  MatrixType=fixdt(1,32,20)  MatrixSize=[1 1]  ColumnIndices=[1]  RowIndices=[1]  PropDataType=fixdt(1,32,19)  defWL=32
  State Out : Outport  VectorParamsAs1DForOutWhenUnconnected=off
  wires:
  Sel/1 -> State Update/2, Bias/1(Sel)
  In1/1 -> Multiply Input/1
  State Update/1 -> State Out/1
  State/1 -> Mux/1
  Bias/1(Out1) -> Mux/2
  Mux/1 -> State Update/1

== system tous/FPGA/HDL Subsystem Boost/HDL Algorithm/Mode Selection/Generate Mode Vector ==
  note: This variant subsystem was automatically generated by the Fixed-Point Tool to convert a MATLAB function block to fixed-point.
      |
      | The variant subsystem contains two blocks:
      | 1. Generate Mode Vector is the original code from the MATLAB function block. Modify this block to update your code or resolve errors.
      |
      | 2. Generate Mode Vector_FixPt is the generated fixed-point code for the MATLAB function block. Any modifications to this block will be overwritten on the next conversion.
      |
      | The Fixed-Point Tool will select an appropriate variant based on the Model Settings. Learn more.
  x : Inport
  u : Inport  Port=2
  t : Inport  Port=3
  Generate Mode Vector : MATLAB Function  TreatAsAtomicUnit=on  VariantControl=false()
  Generate Mode Vector_FixPt : MATLAB Function  TreatAsAtomicUnit=on  VariantControl=(default)
  vs : Outport

== system tous/FPGA/HDL Subsystem Boost/HDL Algorithm/Mode Selection/Output Mode Vector To Index ==
  In1 : Inport
  Index : Constant  Value=fi(0,0,1,0)  SampleTime=2.5e-08  LockScale=on
  Term : Terminator
  Out1 : Outport  VectorParamsAs1DForOutWhenUnconnected=off
  wires:
  In1/1 -> Term/1
  Index/1 -> Out1/1

== system tous/FPGA/HDL Subsystem Boost/HDL Algorithm/Output/Bias ==
  Sel : Inport  LockScale=on
  Bias : Constant  Value=single(stateSpaceParameters_1.Y0d)  OutDataTypeStr=fixdt(1,32,27)  SampleTime=2.5e-08
  Terminator : Terminator
  Out1 : Outport  VectorParamsAs1DForOutWhenUnconnected=off
  wires:
  Sel/1 -> Terminator/1
  Bias/1 -> Out1/1

== system tous/FPGA/HDL Subsystem Boost/HDL Algorithm/State Update/Bias ==
  Sel : Inport  LockScale=on
  Bias : Constant  Value=single(reshape(stateSpaceParameters_1.F0d,4,4))  OutDataTypeStr=fixdt(1,32,27)  SampleTime=2.5e-08
  Data Type Conversion : DataTypeConversion  OutDataTypeStr=uint32  RndMeth=Nearest  SaturateOnIntegerOverflow=off
  Reshape : Reshape
  Selector : Selector  NumberOfDimensions=2  IndexMode=Zero-based  InputPortWidth=3  IndexOptions=Select all,Index vector (port)  Indices=[1 3]  OutputSizes=1
  Out1 : Outport  VectorParamsAs1DForOutWhenUnconnected=off
  wires:
  Selector/1 -> Reshape/1
  Bias/1 -> Selector/1
  Sel/1 -> Data Type Conversion/1
  Data Type Conversion/1 -> Selector/2
  Reshape/1 -> Out1/1

== system tous/FPGA/HDL Subsystem Buck/HDL Algorithm/Mode Selection/Generate Mode Vector ==
  note: This variant subsystem was automatically generated by the Fixed-Point Tool to convert a MATLAB function block to fixed-point.
      |
      | The variant subsystem contains two blocks:
      | 1. Generate Mode Vector is the original code from the MATLAB function block. Modify this block to update your code or resolve errors.
      |
      | 2. Generate Mode Vector_FixPt is the generated fixed-point code for the MATLAB function block. Any modifications to this block will be overwritten on the next conversion.
      |
      | The Fixed-Point Tool will select an appropriate variant based on the Model Settings. Learn more.
  x : Inport
  u : Inport  Port=2
  t : Inport  Port=3
  Generate Mode Vector : MATLAB Function  TreatAsAtomicUnit=on  VariantControl=false()
  Generate Mode Vector_FixPt : MATLAB Function  TreatAsAtomicUnit=on  VariantControl=(default)
  vs : Outport

== system tous/FPGA/HDL Subsystem Buck/HDL Algorithm/Mode Selection/Output Mode Vector To Index ==
  In1 : Inport
  Index : Constant  Value=fi(0,0,1,0)  SampleTime=2.5e-08  LockScale=on
  Term : Terminator
  Out1 : Outport  VectorParamsAs1DForOutWhenUnconnected=off
  wires:
  In1/1 -> Term/1
  Index/1 -> Out1/1

== system tous/FPGA/HDL Subsystem Buck/HDL Algorithm/Output/Bias ==
  Sel : Inport  LockScale=on
  Bias : Constant  Value=single(stateSpaceParameters_1.Y0d)  OutDataTypeStr=fixdt(1,32,24)  SampleTime=2.5e-08
  Terminator : Terminator
  Out1 : Outport  VectorParamsAs1DForOutWhenUnconnected=off
  wires:
  Sel/1 -> Terminator/1
  Bias/1 -> Out1/1

== system tous/FPGA/HDL Subsystem Buck/HDL Algorithm/State Update/Bias ==
  Sel : Inport  LockScale=on
  Bias : Constant  Value=single(reshape(stateSpaceParameters_1.F0d,5,4))  OutDataTypeStr=fixdt(1,32,24)  SampleTime=2.5e-08
  Data Type Conversion : DataTypeConversion  OutDataTypeStr=uint32  RndMeth=Nearest  SaturateOnIntegerOverflow=off
  Reshape : Reshape
  Selector : Selector  NumberOfDimensions=2  IndexMode=Zero-based  InputPortWidth=3  IndexOptions=Select all,Index vector (port)  Indices=[1 3]  OutputSizes=1
  Out1 : Outport  VectorParamsAs1DForOutWhenUnconnected=off
  wires:
  Selector/1 -> Reshape/1
  Bias/1 -> Selector/1
  Sel/1 -> Data Type Conversion/1
  Data Type Conversion/1 -> Selector/2
  Reshape/1 -> Out1/1

== system tous/FPGA/HDL Subsystem Buck-Boost/HDL Algorithm/Mode Selection/Generate Mode Vector ==
  note: This variant subsystem was automatically generated by the Fixed-Point Tool to convert a MATLAB function block to fixed-point.
      |
      | The variant subsystem contains two blocks:
      | 1. Generate Mode Vector is the original code from the MATLAB function block. Modify this block to update your code or resolve errors.
      |
      | 2. Generate Mode Vector_FixPt is the generated fixed-point code for the MATLAB function block. Any modifications to this block will be overwritten on the next conversion.
      |
      | The Fixed-Point Tool will select an appropriate variant based on the Model Settings. Learn more.
  x : Inport
  u : Inport  Port=2
  t : Inport  Port=3
  Generate Mode Vector : MATLAB Function  TreatAsAtomicUnit=on  VariantControl=false()
  Generate Mode Vector_FixPt : MATLAB Function  TreatAsAtomicUnit=on  VariantControl=(default)
  vs : Outport

== system tous/FPGA/HDL Subsystem Buck-Boost/HDL Algorithm/Mode Selection/Output Mode Vector To Index ==
  In1 : Inport
  Index : Constant  Value=fi(0,0,1,0)  SampleTime=2.5e-08  LockScale=on
  Term : Terminator
  Out1 : Outport  VectorParamsAs1DForOutWhenUnconnected=off
  wires:
  In1/1 -> Term/1
  Index/1 -> Out1/1

== system tous/FPGA/HDL Subsystem Buck-Boost/HDL Algorithm/Output/Bias ==
  Sel : Inport  LockScale=on
  Bias : Constant  Value=single(stateSpaceParameters_1.Y0d)  OutDataTypeStr=fixdt(1,32,25)  SampleTime=2.5e-08
  Terminator : Terminator
  Out1 : Outport  VectorParamsAs1DForOutWhenUnconnected=off
  wires:
  Sel/1 -> Terminator/1
  Bias/1 -> Out1/1

== system tous/FPGA/HDL Subsystem Buck-Boost/HDL Algorithm/State Update/Bias ==
  Sel : Inport  LockScale=on
  Bias : Constant  Value=single(reshape(stateSpaceParameters_1.F0d,4,4))  OutDataTypeStr=fixdt(1,32,25)  SampleTime=2.5e-08
  Data Type Conversion : DataTypeConversion  OutDataTypeStr=uint32  RndMeth=Nearest  SaturateOnIntegerOverflow=off
  Reshape : Reshape
  Selector : Selector  NumberOfDimensions=2  IndexMode=Zero-based  InputPortWidth=3  IndexOptions=Select all,Index vector (port)  Indices=[1 3]  OutputSizes=1
  Out1 : Outport  VectorParamsAs1DForOutWhenUnconnected=off
  wires:
  Selector/1 -> Reshape/1
  Bias/1 -> Selector/1
  Sel/1 -> Data Type Conversion/1
  Data Type Conversion/1 -> Selector/2
  Reshape/1 -> Out1/1

== matlab function tous/FPGA/HDL Subsystem Buck/HDL Algorithm/Mode Selection/Generate Mode Vector/Generate Mode Vector ==
  settings: fimath=fimath('RoundingMethod', 'Floor','OverflowAction', 'Wrap','ProductMode', 'FullPrecision', 'SumMode', 'FullPrecision')
  data: x input; u input; vs output; t input
function vs = compute_modes(x, u, t)

  tmp1 = ((-1.0) .* x(3));
  tmp2 = u(1);

  v1 = (tmp1 > (0.7));
  v2 = (tmp2 > (2.0));

  vs = [v1 v2];

end

== matlab function tous/FPGA/HDL Subsystem Boost/HDL Algorithm/Mode Selection/Generate Mode Vector/Generate Mode Vector ==
  data: x input; u input; vs output; t input
function vs = compute_modes(x, u, t)

  tmp1 = (((-1.0) .* x(1)) + ((-1e-06) .* x(3)) + ((-1.0) .* x(4)) + (5.0));
  tmp2 = u(1);

  v1 = (tmp1 > (0.7));
  v2 = (tmp2 > (2.0));

  vs = [v1 v2];

end

== matlab function tous/FPGA/HDL Subsystem Boost/HDL Algorithm/Mode Selection/Generate Mode Vector/Generate Mode Vector_FixPt ==
  settings: fimath=fimath('RoundingMethod', 'Floor', 'OverflowAction', 'Wrap', 'ProductMode', 'FullPrecision', 'MaxProductWordLength', 128, 'SumMode', 'FullPrecision', 'MaxSumWordLength', 128)
  data: x input; u input; vs output; t input
%auto-generated
%#codegen
function vs = compute_modes_fixpt(x, u, t)

  fm = get_fimath();
  u = fi(u, 0, 32, 29, fm);

  tmp1 = (((fi(-1.0, 1, 2, 0, fm)) .* x(1)) + ((fi(-1e-06, 1, 16, 34, fm)) .* x(3)) + ((fi(-1.0, 1, 2, 0, fm)) .* x(4)) + (fi(5.0, 0, 3, 0, fm)));
  tmp2 = fi(u(1), 0, 32, 29, fm);

  v1 = (tmp1 > (fi(0.7, 0, 16, 16, fm)));
  v2 = (tmp2 > (fi(2.0, 0, 2, 0, fm)));

  vs = [v1 v2];

end


function fm = get_fimath()
	fm = fimath('RoundingMethod', 'Floor',...
	     'OverflowAction', 'Wrap',...
	     'ProductMode','FullPrecision',...
	     'MaxProductWordLength', 128,...
	     'SumMode','FullPrecision',...
	     'MaxSumWordLength', 128);
end

== matlab function tous/FPGA/HDL Subsystem Buck-Boost/HDL Algorithm/Mode Selection/Generate Mode Vector/Generate Mode Vector ==
  data: x input; u input; vs output; t input
function vs = compute_modes(x, u, t)

  tmp1 = (x(1) + ((1e-06) .* x(3)) + ((-1.0) .* x(4)));
  tmp2 = u(1);

  v1 = (tmp1 > (0.7));
  v2 = (tmp2 > (2.0));

  vs = [v1 v2];

end

== matlab function tous/FPGA/HDL Subsystem Buck-Boost/HDL Algorithm/Mode Selection/Generate Mode Vector/Generate Mode Vector_FixPt ==
  settings: fimath=fimath('RoundingMethod', 'Floor', 'OverflowAction', 'Wrap', 'ProductMode', 'FullPrecision', 'MaxProductWordLength', 128, 'SumMode', 'FullPrecision', 'MaxSumWordLength', 128)
  data: x input; u input; vs output; t input
%auto-generated
%#codegen
function vs = compute_modes_fixpt(x, u, t)

  fm = get_fimath();
  u = fi(u, 0, 32, 29, fm);

  tmp1 = (x(1) + ((fi(1e-06, 0, 16, 35, fm)) .* x(3)) + ((fi(-1.0, 1, 2, 0, fm)) .* x(4)));
  tmp2 = fi(u(1), 0, 32, 29, fm);

  v1 = (tmp1 > (fi(0.7, 0, 16, 16, fm)));
  v2 = (tmp2 > (fi(2.0, 0, 2, 0, fm)));

  vs = [v1 v2];

end


function fm = get_fimath()
	fm = fimath('RoundingMethod', 'Floor',...
	     'OverflowAction', 'Wrap',...
	     'ProductMode','FullPrecision',...
	     'MaxProductWordLength', 128,...
	     'SumMode','FullPrecision',...
	     'MaxSumWordLength', 128);
end
